simulink model "LKA"  (R2024a)
settings: Solver=ode1  StartTime=0.0  StopTime=70  FixedStep=1e-1  RelTol=1e-3
model workspace (MAT data in the model file):
  firstWarning = 1
  originalScenarioChecksum = '148AF3F4C6D12E297BC90CA3DB8BB877'
values from neighbouring files (symbols this model uses):
  dt = 0.1    [Parameters.m]
  Ki = 1    [Parameters.m]
  Kp = 1.1    [Parameters.m]
  L1 = 3.7    [Parameters.m]
  lane_width = 3.6    [Parameters.m]
  lr = 1.6    [Parameters.m]
  m = 1575    [Parameters.m]
  PredictionHorizon = 2    [Parameters.m]
  tau1 = 0.5    [Parameters.m]
  tau2 = 0.07    [Parameters.m]
undefined symbols (not defined in the file or in its folder): driving
libraries: drivingscenarioandsensors x2, simulink x2, simulink_extras x2, slpidlib x1, autolibshared x1
settings Model: Creator=apple  LastModifiedBy=apple
settings OptimizationCC: DefaultParameterBehavior=Inlined  UseDivisionForNetSlopeComputation=on  GainParamInheritBuiltInType=on  UseFloatMulNetSlope=on  InlineInvariantSignals=on  PassReuseOutputArgsAs=Individual arguments  ZeroExternalMemoryAtStartup=off  ZeroInternalMemoryAtStartup=off  NoFixptDivByZeroProtection=on  EfficientFloat2IntCast=on  LifeSpan=1  OptimizeBlockOrder=speed  DifferentSizesBufferReuse=on  EfficientTunableParamExpr=on
settings DebuggingCC: ParameterTunabilityLossMsg=error
settings HardwareCC: ProdBitPerLong=64  ProdLongLongMode=on  ProdHWDeviceType=Apple->ARM64
settings SFSimCC: MATLABDynamicMemAlloc=off
settings RTWCC: Description=Embedded Coder  SystemTargetFile=ert.tlc  TemplateMakefile=ert_default_tmf
settings CodeAppCC: ForceParamTrailComments=on  IgnoreCustomStorageClasses=off  OperatorAnnotations=on  SimulinkDataObjDesc=on  SFDataObjDesc=on  CustomSymbolStrGlobalVar=rt$N$M  CustomSymbolStrType=$N$M  CustomSymbolStrFcn=$N$M$F  CustomSymbolStrMacro=$N$M  InsertBlockDesc=on
settings ERTTargetCC: TargetLangStandard=C99 (ISO)  GenerateSampleERTMain=on  IncludeMdlTerminateFcn=off  CombineSignalStateStructs=on  SupportAbsoluteTime=off  SupportComplex=off  SupportContinuousTime=on  SupportNonInlinedSFcns=on  InlinedParameterPlacement=NonHierarchical  ERTCustomFileTemplate=example_file_process.tlc  ERTFilePackagingFormat=CompactWithDataFile
settings ConfigComp: DVTestSuiteOptimization=Auto  DVDetectOutOfBounds=on  DVModelReferenceHarness=on  DVHarnessSource=Signal Editor

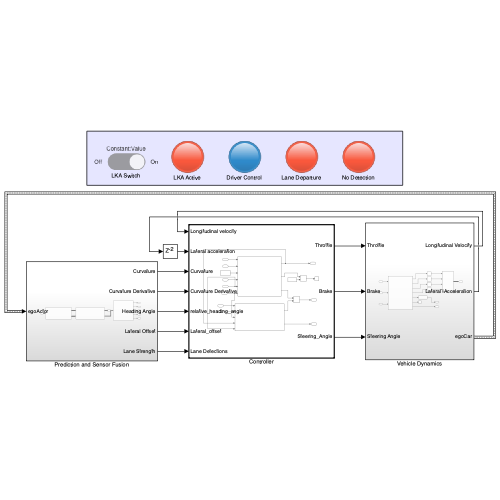
[thumbnail: Simulink's stored preview of the top-level diagram]
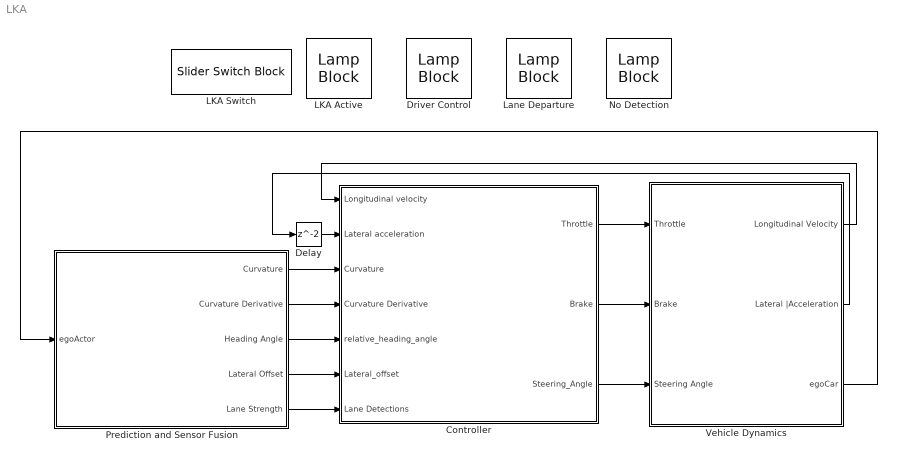
== system LKA ==
  Controller : Subsystem  TreatAsAtomicUnit=on
  Delay : Delay
  Driver Control : LampBlock  LabelPosition=Hide
  LKA Active : LampBlock  LabelPosition=Hide
  LKA Switch : SliderSwitchBlock
      settings: Values={{'Off', 'On'}, [0 1]}
  Lane Departure : LampBlock  LabelPosition=Hide
  No Detection : LampBlock  LabelPosition=Hide
  Prediction and Sensor Fusion : Subsystem
  Vehicle Dynamics : Subsystem
  wires:
  Vehicle Dynamics/3(egoCar) -> Prediction and Sensor Fusion/1(egoActor)
  Controller/1(Throttle) -> Vehicle Dynamics/1(Throttle)
  Controller/2(Brake) -> Vehicle Dynamics/2(Brake)
  Controller/3(Steering_Angle) -> Vehicle Dynamics/3(Steering Angle)
  Vehicle Dynamics/1(Longitudinal Velocity) -> Controller/1(Longitudinal velocity)
  Vehicle Dynamics/2(Lateral |Acceleration) -> Delay/1
  Prediction and Sensor Fusion/1(Curvature) -> Controller/3(Curvature)
  Prediction and Sensor Fusion/2(Curvature Derivative) -> Controller/4(Curvature Derivative)
  Prediction and Sensor Fusion/3(Heading Angle) -> Controller/5(relative_heading_angle)
  Prediction and Sensor Fusion/4(Lateral Offset) -> Controller/6(Lateral_offset)
  Prediction and Sensor Fusion/5(Lane Strength) -> Controller/7(Lane Detections)
  Delay/1 -> Controller/2(Lateral acceleration)

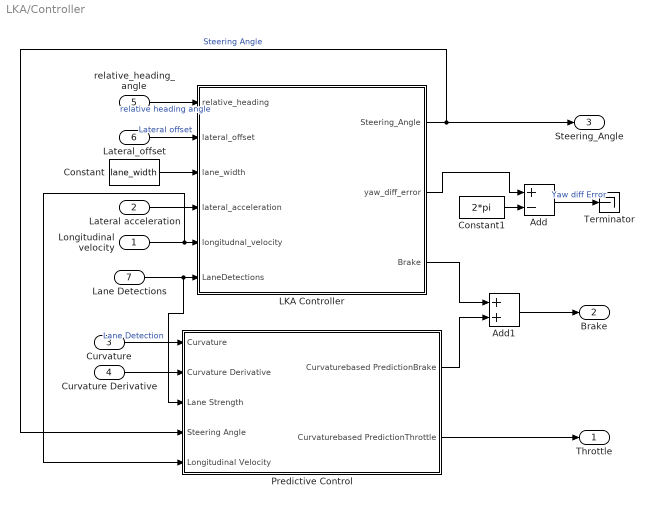
== system LKA/Controller ==
  Longitudinal velocity : Inport
  Lateral acceleration : Inport  Port=2
  Curvature : Inport  Port=3
  Curvature Derivative : Inport  Port=4
  relative_heading_angle : Inport  Port=5
  Lateral_offset : Inport  Port=6
  Lane Detections : Inport  Port=7
  Add : Sum  Inputs=+-
  Add1 : Sum
  Constant : Constant  Value=lane_width
  Constant1 : Constant  Value=2*pi
  LKA Controller : Subsystem
  Predictive Control : Subsystem
  Terminator : Terminator
  Throttle : Outport
  Brake : Outport  Port=2
  Steering_Angle : Outport  Port=3
  wires:
  Constant/1 -> LKA Controller/3(lane_width)
  Lane Detections/1 -> Predictive Control/3(Lane Strength), LKA Controller/6(LaneDetections)  "Lane Detection"
  Lateral acceleration/1 -> LKA Controller/4(lateral_acceleration)
  Lateral_offset/1 -> LKA Controller/2(lateral_offset)  "Lateral offset"
  relative_heading_angle/1 -> LKA Controller/1(relative_heading)  "relative heading angle"
  Longitudinal velocity/1 -> Predictive Control/5(Longitudinal Velocity), LKA Controller/5(longitudnal_velocity)
  LKA Controller/1(Steering_Angle) -> Steering_Angle/1, Predictive Control/4(Steering Angle)  "Steering Angle"
  LKA Controller/2(yaw_diff_error) -> Add/1
  Add/1 -> Terminator/1  "Yaw diff Error"
  Constant1/1 -> Add/2
  Curvature/1 -> Predictive Control/1(Curvature)
  Curvature Derivative/1 -> Predictive Control/2(Curvature Derivative)
  LKA Controller/3(Brake) -> Add1/1
  Predictive Control/1(Curvaturebased PredictionBrake) -> Add1/2
  Add1/1 -> Brake/1
  Predictive Control/2(Curvaturebased PredictionThrottle) -> Throttle/1

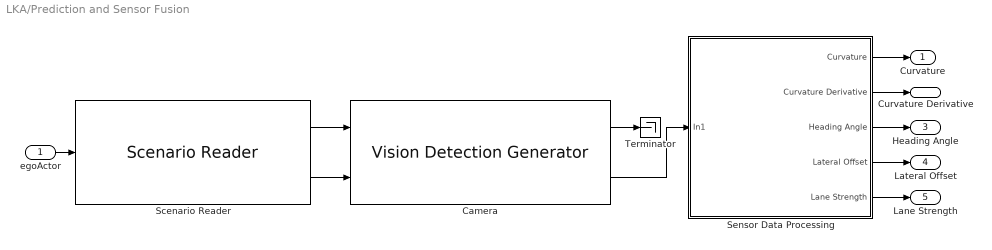
== system LKA/Prediction and Sensor Fusion ==
  egoActor : Inport
  Camera : drivingscenarioandsensors/Vision Detection Generator  SensorIndex=1  DetectorOutput=Lanes and objects  UpdateInterval=dt  LaneUpdateInterval=dt  SensorLocation=[1.9 0]  Height=1.1  Yaw=0  Pitch=10  Roll=0  BusNameSource=Auto  BusName=BusObjectDetections  BusName2Source=Property  BusName2=BusVision  MaxNumDetectionsSource=Property  MaxNumDetections=50  MaxNumLanesSource=Property  MaxNumLanes=2  DetectionCoordinates=Ego Cartesian  SimulateUsing=Interpreted execution  MaxRange=60  BoundingBoxAccuracy=5  ProcessNoiseIntensity=5  MaxSpeed=100  MaxAllowedOcclusion=0.5  MinObjectImageSize=[15 15]  DetectionProbability=0.9  FalsePositivesPerImage=0.1  MinLaneImageSize=[20 3]  LaneBoundaryAccuracy=3  HasNoise=on  InitialSeedSource=Repeatable  InitialSeed=0  UsedSeed=0  ActorProfilesSource=From Scenario Reader block  ActorProfilesParameters=driving.internal.ActorProfilesParameters  ActorProfilesExpression=[struct('ActorID',1,'ClassID',1,'Length',4.7,'Width',1.8,'Height',1.4,'OriginOffset',[-1.35 0 0],'MeshVertices',[3.7 0.9 0.857439446366782;3.7 -0.9 0.857439446366782;3.7 -0.9 0.314878892733564;3.7 0.9 0.314878892733564;3.7 0.9 0.857439446366782;2.525 0.9 0.993079584775086;2.525 -0.9 0.993079584775086;3.7 -0.9 0.857439446366782;1.82 0.72 1.4;0.41 0.72 1.4;0.41 -0.72 1.4;1.82 -0.72 1.4;-0.295 0.9 0.993079584775086;-1 0.9 0.857439446366782;-1 -0.9 0.857439446366782;-0.295 -0.9 0.993079584775086;3.7 0.9 0.857439446366782;3.7 0.9 0.314878892733564;2.525 0.9 0.314878892733564;2.525 0.9 0.993079584775086;2.525 0.9 0.993079584775086;2.525 0.9 0.314878892733564;-0.295 0.9 0.314878892733564;-0.295 0.9 0.993079584775086;-0.295 0.9 0.993079584775086;-0.295 0.9 0.314878892733564;-1 0.9 0.355570934256055;-1 0.9 0.857439446366782;2.525 0.9 0.993079584775086;-0.295 0.9 0.993079584775086;0.41 0.72 1.4;1.82 0.72 1.4;3.7 -0.9 0.857439446366782;3.7 -0.9 0.314878892733564;2.525 -0.9 0.314878892733564;2.525 -0.9 0.993079584775086;2.525 -0.9 0.993079584775086;2.525 -0.9 0.314878892733564;-0.295 -0.9 0.314878892733564;-0.295 -0.9 0.993079584775086;-0.295 -0.9 0.993079584775086;-0.295 -0.9 0.314878892733564;-1 -0.9 0.355570934256055;-1 -0.9 0.857439446366782;2.525 -0.9 0.993079584775086;-0.295 -0.9 0.993079584775086;0.41 -0.72 1.4;1.82 -0.72 1.4;-0.295 0.9 0.993079584775086;-0.295 -0.9 0.993079584775086;0.41 -0.72 1.4;0.41 0.72 1.4;2.525 -0.9 0.993079584775086;1.82 -0.72 1.4;1.82 0.72 1.4;2.525 0.9 0.993079584775086;-1 0.9 0.857439446366782;-1 0.9 0.355570934256055;-1 -0.9 0.355570934256055;-1 -0.9 0.857439446366782;3.7 0.9 0.314878892733564;3.7 -0.9 0.314878892733564;-0.295 -0.9 0.314878892733564;-0.295 0.9 0.314878892733564;-0.295 0.9 0.314878892733564;-1 0.9 0.355570934256055;-1 -0.9 0.355570934256055;-0.295 -0.9 0.314878892733564;0 -0.63 0;0 -0.87 0;0.191030206995054 -0.63 0.0601365173421445;0.191030206995054 -0.87 0.0601365173421445;0.309093367795925 -0.63 0.217575963708927;0.309093367795925 -0.87 0.217575963708927;0.309093367795925 -0.63 0.412181821758201;0.309093367795925 -0.87 0.412181821758201;0.191030206995054 -0.63 0.569621268124983;0.191030206995054 -0.87 0.569621268124983;0 -0.63 0.629757785467128;0 -0.87 0.629757785467128;-0.191030206995054 -0.63 0.569621268124983;-0.191030206995054 -0.87 0.569621268124983;-0.309093367795925 -0.63 0.412181821758201;-0.309093367795925 -0.87 0.412181821758201;-0.309093367795925 -0.63 0.217575963708927;-0.309093367795925 -0.87 0.217575963708927;-0.191030206995054 -0.63 0.0601365173421445;-0.191030206995054 -0.87 0.0601365173421445;0 -0.63 0;0 -0.87 0;0 -0.63 0;0.191030206995054 -0.63 0.0601365173421445;0.309093367795925 -0.63 0.217575963708927;0.309093367795925 -0.63 0.412181821758201;0.191030206995054 -0.63 0.569621268124983;0 -0.63 0.629757785467128;-0.191030206995054 -0.63 0.569621268124983;-0.309093367795925 -0.63 0.412181821758201;-0.309093367795925 -0.63 0.217575963708927;-0.191030206995054 -0.63 0.0601365173421445;0 -0.87 0;0.191030206995054 -0.87 0.0601365173421445;0.309093367795925 -0.87 0.217575963708927;0.309093367795925 -0.87 0.412181821758201;0.191030206995054 -0.87 0.569621268124983;0 -0.87 0.629757785467128;-0.191030206995054 -0.87 0.569621268124983;-0.309093367795925 -0.87 0.412181821758201;-0.309093367795925 -0.87 0.217575963708927;-0.191030206995054 -0.87 0.0601365173421445;0 0.87 0;0 0.63 0;0.191030206995054 0.87 0.0601365173421445;0.191030206995054 0.63 0.0601365173421445;0.309093367795925 0.87 0.217575963708927;0.309093367795925 0.63 0.217575963708927;0.309093367795925 0.87 0.412181821758201;0.309093367795925 0.63 0.412181821758201;0.191030206995054 0.87 0.569621268124983;0.191030206995054 0.63 0.569621268124983;0 0.87 0.629757785467128;0 0.63 0.629757785467128;-0.191030206995054 0.87 0.569621268124983;-0.191030206995054 0.63 0.569621268124983;-0.309093367795925 0.87 0.412181821758201;-0.309093367795925 0.63 0.412181821758201;-0.309093367795925 0.87 0.217575963708927;-0.309093367795925 0.63 0.217575963708927;-0.191030206995054 0.87 0.0601365173421445;-0.191030206995054 0.63 0.0601365173421445;0 ...(+3718 chars)],'MeshFaces',[1 2 3;3 4 1;5 6 7;7 8 5;9 10 11;11 12 9;13 14 15;15 16 13;17 18 19;19 20 17;21 22 23;23 24 21;25 26 27;27 28 25;29 30 31;31 32 29;33 34 35;35 36 33;37 38 39;39 40 37;41 42 43;43 44 41;45 46 47;47 48 45;49 50 51;51 52 49;53 54 55;55 56 53;57 58 59;59 60 57;61 62 63;63 64 61;65 66 67;67 68 65;69 71 72;72 70 69;71 73 74;74 72 71;73 75 76;76 74 73;75 77 78;78 76 75;77 79 80;80 78 77;79 81 82;82 80 79;81 83 84;84 82 81;83 85 86;86 84 83;85 87 88;88 86 85;87 89 90;90 88 87;91 92 93;91 93 94;91 94 95;91 95 96;91 96 97;91 97 98;91 98 99;91 99 100;101 102 103;101 103 104;101 104 105;101 105 106;101 106 107;101 107 108;101 108 109;101 109 110;111 113 114;114 112 111;113 115 116;116 114 113;115 117 118;118 116 115;117 119 120;120 118 117;119 121 122;122 120 119;121 123 124;124 122 121;123 125 126;126 124 123;125 127 128;128 126 125;127 129 130;130 128 127;129 131 132;132 130 129;133 134 135;133 135 136;133 136 137;133 137 138;133 138 139;133 139 140;133 140 141;133 141 142;143 144 145;143 145 146;143 146 147;143 147 148;143 148 149;143 149 150;143 150 151;143 151 152;153 155 156;156 154 153;155 157 158;158 156 155;157 159 160;160 158 157;159 161 162;162 160 159;161 163 164;164 162 161;163 165 166;166 164 163;165 167 168;168 166 165;167 169 170;170 168 167;169 171 172;172 170 169;171 173 174;174 172 171;175 176 177;175 177 178;175 178 179;175 179 180;175 180 181;175 181 182;175 182 183;175 183 184;185 186 187;185 187 188;185 188 189;185 189 190;185 190 191;185 191 192;185 192 193;185 193 194;195 197 198;198 196 195;197 199 200;200 198 197;199 201 202;202 200 199;201 203 204;204 202 201;203 205 206;206 204 203;205 207 208;208 206 205;207 209 210;210 208 207;209 211 212;212 210 209;211 213 214;214 212 211;213 215 216;216 214 213;217 218 219;217 219 220;217 220 221;217 221 222;217 222 223;217 223 224;217 224 225;217 225 226;227 228 229;227 229 230;227 230 231;227 231 232;227 232 233;227 233 234;227 234 235;227 235 236],'RCSPattern',[10 10;10 10],'RCSAzimuthAngles',[-180 180],'RCSElevationAngles',[-90 90])]  Intrinsics=driving.internal.cameraIntrinsics('FocalLength',[340 720],'PrincipalPoint',[640 480],'ImageSize',[960 1280],'RadialDistortion',[0 0],'TangentialDistortion',[0 0],'Skew',0)
  Scenario Reader : drivingscenarioandsensors/Scenario Reader  ScenarioSource=From file  ScenarioFileName=/Users/apple/Documents/VCSE/Practice/test_scenario_1.mat  ScenarioVariableName=scenario  OutputCoordinateSystem=Vehicle coordinates  EgoVehicleSource=Input port  EgoVehicleActorID=1  OrientVehiclesOnRoad=off  OutputEgoVehiclePose=off  OutputEgoVehicleState=off  SampleTime=dt  LaneBoundaryOutput=Ego vehicle lane boundaries  LaneBoundaryDistance=0:0.5:60  LaneBoundaryLocation=Inner edge of lane markings  BusNameSource=Auto  BusName=BusActors  BusNumActorsSource=Scenario  BusNumActors=100  BusName2Source=Auto  BusName2=BusLaneBoundaries  BusNumLaneBoundariesSource=Scenario  BusNumLaneBoundaries=10  BusName3Source=Auto  BusName3=BusEgoActor  BusName4Source=Auto  BusName4=BusEgoState  ShowCoordinateLabels=on  SimulateUsing=Interpreted execution
  Sensor Data Processing : Subsystem
  Terminator : Terminator
  Curvature : Outport
  Curvature Derivative : Outport  Port=2
  Heading Angle : Outport  Port=3
  Lateral Offset : Outport  Port=4
  Lane Strength : Outport  Port=5
  wires:
  Camera/1 -> Terminator/1
  Scenario Reader/2 -> Camera/2
  Camera/2 -> Sensor Data Processing/1(In1)
  egoActor/1 -> Scenario Reader/1
  Scenario Reader/1 -> Camera/1
  Sensor Data Processing/2(Curvature Derivative) -> Curvature Derivative/1
  Sensor Data Processing/1(Curvature) -> Curvature/1
  Sensor Data Processing/3(Heading Angle) -> Heading Angle/1
  Sensor Data Processing/4(Lateral Offset) -> Lateral Offset/1
  Sensor Data Processing/5(Lane Strength) -> Lane Strength/1

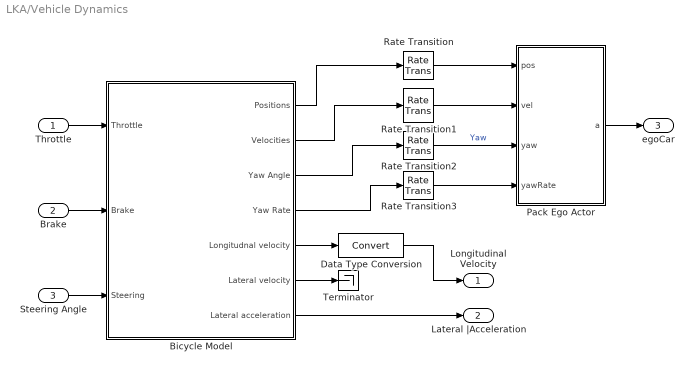
== system LKA/Vehicle Dynamics ==
  Throttle : Inport
  Brake : Inport  Port=2
  Steering Angle : Inport  Port=3
  Bicycle Model : Subsystem
  Data Type Conversion : DataTypeConversion  SaturateOnIntegerOverflow=off  RndMeth=Floor
  Pack Ego Actor : MATLAB Function  TreatAsAtomicUnit=on
  Rate Transition{,1..3} (4 alike) : RateTransition  OutPortSampleTime=Ts
  Terminator : Terminator
  Longitudinal Velocity : Outport
  Lateral |Acceleration : Outport  Port=2
  egoCar : Outport  Port=3
  wires:
  Bicycle Model/1(Positions) -> Rate Transition/1
  Bicycle Model/2(Velocities) -> Rate Transition1/1
  Bicycle Model/3(Yaw Angle) -> Rate Transition2/1
  Bicycle Model/4(Yaw Rate) -> Rate Transition3/1
  Bicycle Model/5(Longitudnal velocity) -> Data Type Conversion/1
  Data Type Conversion/1 -> Longitudinal Velocity/1
  Bicycle Model/6(Lateral velocity) -> Terminator/1
  Bicycle Model/7(Lateral acceleration) -> Lateral |Acceleration/1
  Steering Angle/1 -> Bicycle Model/3(Steering)
  Brake/1 -> Bicycle Model/2(Brake)
  Throttle/1 -> Bicycle Model/1(Throttle)
  Pack Ego Actor/1(a) -> egoCar/1
  Rate Transition/1 -> Pack Ego Actor/1(pos)
  Rate Transition1/1 -> Pack Ego Actor/2(vel)
  Rate Transition2/1 -> Pack Ego Actor/3(yaw)  "Yaw"
  Rate Transition3/1 -> Pack Ego Actor/4(yawRate)

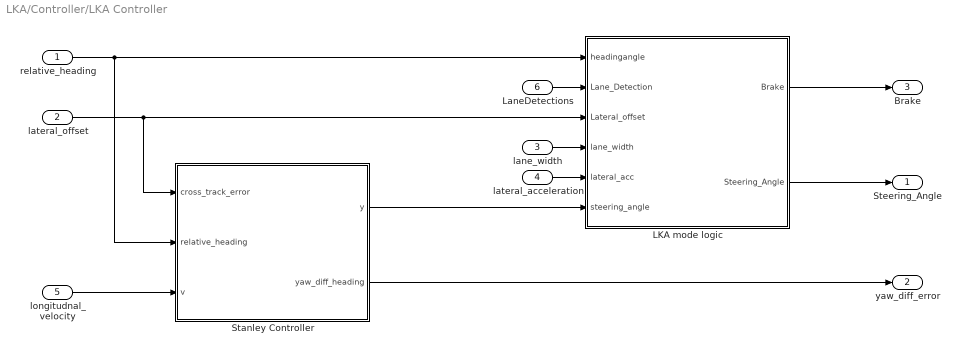
== system LKA/Controller/LKA Controller ==
  relative_heading : Inport
  lateral_offset : Inport  Port=2
  lane_width : Inport  Port=3
  lateral_acceleration : Inport  Port=4
  longitudnal_velocity : Inport  Port=5
  LaneDetections : Inport  Port=6
  LKA mode logic : Subsystem
  Stanley Controller : MATLAB Function  TreatAsAtomicUnit=on
  Steering_Angle : Outport
  yaw_diff_error : Outport  Port=2
  Brake : Outport  Port=3
  wires:
  LKA mode logic/2(Steering_Angle) -> Steering_Angle/1
  LKA mode logic/1(Brake) -> Brake/1
  lateral_acceleration/1 -> LKA mode logic/5(lateral_acc)
  longitudnal_velocity/1 -> Stanley Controller/3(v)
  lateral_offset/1 -> LKA mode logic/3(Lateral_offset), Stanley Controller/1(cross_track_error)
  lane_width/1 -> LKA mode logic/4(lane_width)
  Stanley Controller/1(y) -> LKA mode logic/6(steering_angle)
  LaneDetections/1 -> LKA mode logic/2(Lane_Detection)
  Stanley Controller/2(yaw_diff_heading) -> yaw_diff_error/1
  relative_heading/1 -> LKA mode logic/1(headingangle), Stanley Controller/2(relative_heading)

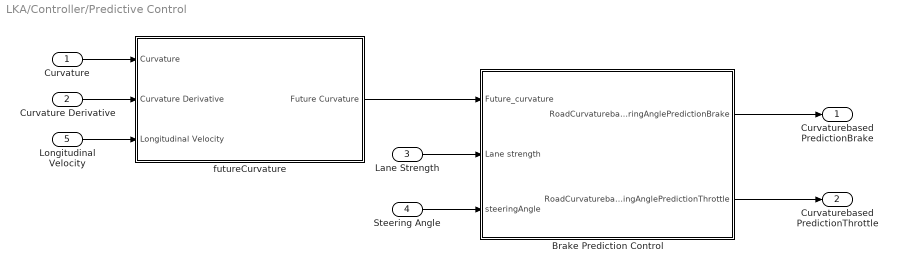
== system LKA/Controller/Predictive Control ==
  Curvature : Inport
  Curvature Derivative : Inport  Port=2
  Lane Strength : Inport  Port=3
  Steering Angle : Inport  Port=4
  Longitudinal Velocity : Inport  Port=5
  Brake Prediction Control : Subsystem
  futureCurvature : Subsystem
  Curvaturebased PredictionBrake : Outport
  Curvaturebased PredictionThrottle : Outport  Port=2
  wires:
  Curvature/1 -> futureCurvature/1(Curvature)
  Curvature Derivative/1 -> futureCurvature/2(Curvature Derivative)
  Longitudinal Velocity/1 -> futureCurvature/3(Longitudinal Velocity)
  futureCurvature/1(Future Curvature) -> Brake Prediction Control/1(Future_curvature)
  Lane Strength/1 -> Brake Prediction Control/2(Lane strength)
  Steering Angle/1 -> Brake Prediction Control/3(steeringAngle)
  Brake Prediction Control/2(RoadCurvaturebased SteeringAnglePredictionThrottle) -> Curvaturebased PredictionThrottle/1
  Brake Prediction Control/1(RoadCurvaturebased SteeringAnglePredictionBrake) -> Curvaturebased PredictionBrake/1

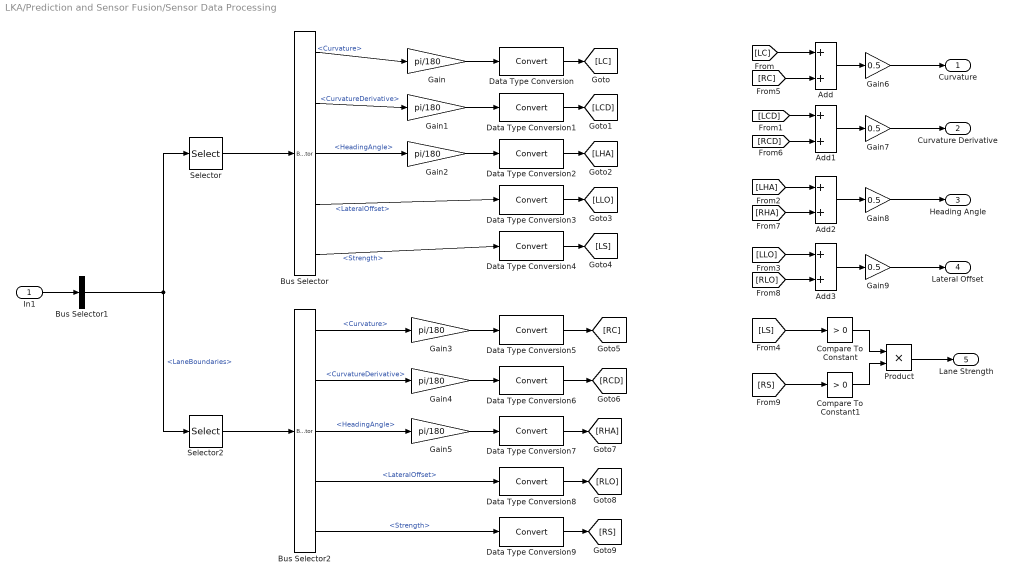
== system LKA/Prediction and Sensor Fusion/Sensor Data Processing ==
  In1 : Inport
  Add{,1..3} (4 alike) : Sum
  Bus Selector : BusSelector  OutputSignals=Curvature,CurvatureDerivative,HeadingAngle,LateralOffset,Strength
  Bus Selector1 : BusSelector  OutputSignals=LaneBoundaries
  Bus Selector2 : BusSelector  OutputSignals=Curvature,CurvatureDerivative,HeadingAngle,LateralOffset,Strength
  Compare To Constant : simulink/Logic and Bit Operations/Compare To Constant  relop=>  const=0  OutDataTypeStr=boolean
  Compare To Constant1 : simulink/Logic and Bit Operations/Compare To Constant  relop=>  const=0  OutDataTypeStr=boolean
  Data Type Conversion{,1..9} (10 alike) : DataTypeConversion  SaturateOnIntegerOverflow=off  RndMeth=Floor
  Gain{,1..5} (6 alike) : Gain  Gain=pi/180
  Gain{6..9} (4 alike) : Gain  Gain=0.5
  Product : Product
  Selector : Selector  InputPortWidth=2  IndexOptions=Index vector (dialog)  Indices=1  OutputSizes=1
  Selector2 : Selector  InputPortWidth=2  IndexOptions=Index vector (dialog)  Indices=2  OutputSizes=1
  Curvature : Outport
  Curvature Derivative : Outport  Port=2
  Heading Angle : Outport  Port=3
  Lateral Offset : Outport  Port=4
  Lane Strength : Outport  Port=5
  wires:
  In1/1 -> Bus Selector1/1
  Bus Selector1/1 -> Selector2/1, Selector/1  "<LaneBoundaries>"
  Selector2/1 -> Bus Selector2/1
  Selector/1 -> Bus Selector/1
  Bus Selector/1 -> Gain/1  "<Curvature>"
  Bus Selector/2 -> Gain1/1  "<CurvatureDerivative>"
  Bus Selector/3 -> Gain2/1  "<HeadingAngle>"
  Bus Selector/4 -> Data Type Conversion3/1  "<LateralOffset>"
  Bus Selector/5 -> Data Type Conversion4/1  "<Strength>"
  Bus Selector2/1 -> Gain3/1  "<Curvature>"
  Gain/1 -> Data Type Conversion/1
  Gain1/1 -> Data Type Conversion1/1
  Gain2/1 -> Data Type Conversion2/1
  Gain4/1 -> Data Type Conversion6/1
  Gain5/1 -> Data Type Conversion7/1
  Bus Selector2/5 -> Data Type Conversion9/1  "<Strength>"
  Gain3/1 -> Data Type Conversion5/1
  Bus Selector2/4 -> Data Type Conversion8/1  "<LateralOffset>"
  Bus Selector2/2 -> Gain4/1  "<CurvatureDerivative>"
  Bus Selector2/3 -> Gain5/1  "<HeadingAngle>"
  Data Type Conversion/1 -> [LC]
  Data Type Conversion2/1 -> [LHA]
  Data Type Conversion1/1 -> [LCD]
  Data Type Conversion3/1 -> [LLO]
  Data Type Conversion4/1 -> [LS]
  Data Type Conversion5/1 -> [RC]
  Data Type Conversion6/1 -> [RCD]
  Data Type Conversion7/1 -> [RHA]
  Data Type Conversion8/1 -> [RLO]
  Data Type Conversion9/1 -> [RS]
  [LC] -> Add/1
  [RC] -> Add/2
  Add/1 -> Gain6/1
  Gain6/1 -> Curvature/1
  Gain7/1 -> Curvature Derivative/1
  Add1/1 -> Gain7/1
  [LCD] -> Add1/1
  [RCD] -> Add1/2
  Gain8/1 -> Heading Angle/1
  Add2/1 -> Gain8/1
  [LHA] -> Add2/1
  [RHA] -> Add2/2
  Gain9/1 -> Lateral Offset/1
  Add3/1 -> Gain9/1
  [LLO] -> Add3/1
  [RLO] -> Add3/2
  [LS] -> Compare To Constant/1
  [RS] -> Compare To Constant1/1
  Compare To Constant1/1 -> Product/2
  Compare To Constant/1 -> Product/1
  Product/1 -> Lane Strength/1

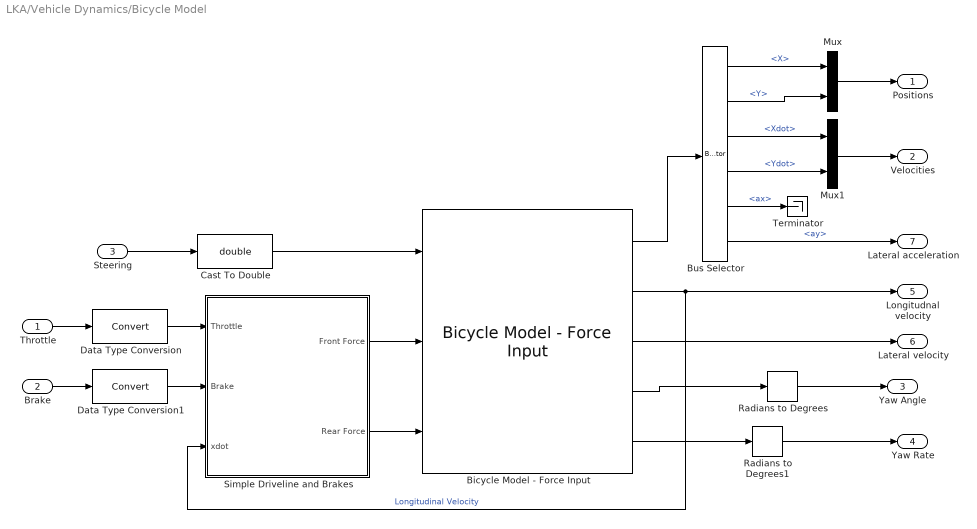
== system LKA/Vehicle Dynamics/Bicycle Model ==
  Throttle : Inport
  Brake : Inport  Port=2
  Steering : Inport  Port=3
  Bicycle Model - Force Input : autolibshared/Bicycle Model - Force Input  trackMode=Single (bicycle)  inputMode=External longitudinal forces  frontSteerMode=on  rearSteerMode=off  windMode=off  muMode=off  extFMode=off  extMMode=off  aMode=3  NF=2  NR=2  m=m  a=lf  b=lr  h=0.35  X_o=x0_ego  xdot_o=v0_ego  CalphaMode=off  sigmaMode=on  w=[1.4,1.4]  Cy_f=Cf  Cy_r=Cr  sigma_f=.1  sigma_r=.1  alpha_f_brk=[-.1 .1]  Cy_f_data=[-9e3 9e3]  alpha_r_brk=[-.1 .1]  Cy_r_data=[-9e3 9e3]  Y_o=y0_ego  ydot_o=0  Izz=Iz  psi_o=0  r_o=yaw0_ego  Af=0  Cd=.3  Cl=.1  Cpm=.1  beta_w=[0:0.01:0.3]  Cs=[0:0.03:0.9]  Cym=[0:0.01:0.3]  Pabs=101325  Tair=273  g=9.81  mu=1  xdot_tol=.01  Fznom=5000  Fxtire_sat=1e6  Fytire_sat=1e6  longOff=0  latOff=0  vertOff=0
      settings: LibrarySourceBlock=drivingscenarioandsensors/Bicycle Model - Force Input
  Bus Selector : BusSelector  OutputSignals=InertFrm.FrntAxl.Disp.X,InertFrm.FrntAxl.Disp.Y,InertFrm.FrntAxl.Vel.Xdot,InertFrm.FrntAxl.Vel.Ydot,BdyFrm.Cg.Acc.ax,BdyFrm.Cg.Acc.ay
  Cast To Double : DataTypeConversion  OutDataTypeStr=double  SaturateOnIntegerOverflow=off  RndMeth=Floor
  Data Type Conversion : DataTypeConversion  SaturateOnIntegerOverflow=off  RndMeth=Floor
  Data Type Conversion1 : DataTypeConversion  SaturateOnIntegerOverflow=off  RndMeth=Floor
  Mux : Mux  Inputs=2
  Mux1 : Mux  Inputs=2
  Radians to Degrees : simulink_extras/Transformations/Radians to Degrees
  Radians to Degrees1 : simulink_extras/Transformations/Radians to Degrees
  Simple Driveline and Brakes : Subsystem
  Terminator : Terminator
  Positions : Outport
  Velocities : Outport  Port=2
  Yaw Angle : Outport  Port=3
  Yaw Rate : Outport  Port=4
  Longitudnal velocity : Outport  Port=5
  Lateral velocity : Outport  Port=6
  Lateral acceleration : Outport  Port=7
  wires:
  Steering/1 -> Cast To Double/1
  Cast To Double/1 -> Bicycle Model - Force Input/1
  Simple Driveline and Brakes/1(Front Force) -> Bicycle Model - Force Input/2
  Simple Driveline and Brakes/2(Rear Force) -> Bicycle Model - Force Input/3
  Throttle/1 -> Data Type Conversion/1
  Brake/1 -> Data Type Conversion1/1
  Data Type Conversion1/1 -> Simple Driveline and Brakes/2(Brake)
  Data Type Conversion/1 -> Simple Driveline and Brakes/1(Throttle)
  Bicycle Model - Force Input/1 -> Bus Selector/1
  Bus Selector/4 -> Mux1/2  "<Ydot>"
  Bus Selector/6 -> Lateral acceleration/1  "<ay>"
  Bus Selector/5 -> Terminator/1  "<ax>"
  Bus Selector/3 -> Mux1/1  "<Xdot>"
  Bus Selector/2 -> Mux/2  "<Y>"
  Bus Selector/1 -> Mux/1  "<X>"
  Mux/1 -> Positions/1
  Mux1/1 -> Velocities/1
  Bicycle Model - Force Input/2 -> Simple Driveline and Brakes/3(xdot), Longitudnal velocity/1  "Longitudinal Velocity"
  Bicycle Model - Force Input/3 -> Lateral velocity/1
  Bicycle Model - Force Input/5 -> Radians to Degrees1/1
  Radians to Degrees1/1 -> Yaw Rate/1
  Bicycle Model - Force Input/4 -> Radians to Degrees/1
  Radians to Degrees/1 -> Yaw Angle/1

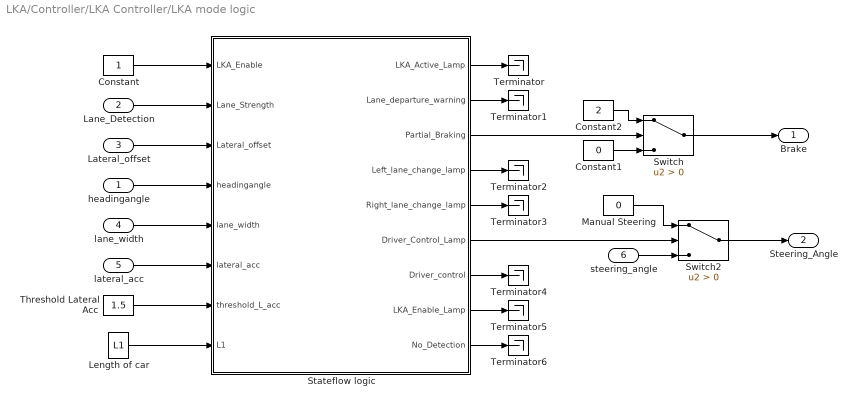
== system LKA/Controller/LKA Controller/LKA mode logic ==
  headingangle : Inport
  Lane_Detection : Inport  Port=2
  Lateral_offset : Inport  Port=3
  lane_width : Inport  Port=4
  lateral_acc : Inport  Port=5
  steering_angle : Inport  Port=6
  Constant : Constant
  Constant1 : Constant  Value=0
  Constant2 : Constant  Value=2
  Length of car : Constant  Value=L1
  Manual Steering : Constant  Value=0
  Stateflow logic : Stateflow chart  TreatAsAtomicUnit=on
  Switch : Switch  Criteria=u2 > Threshold  SaturateOnIntegerOverflow=off  InputSameDT=off
  Switch2 : Switch  Criteria=u2 > Threshold  SaturateOnIntegerOverflow=off  InputSameDT=off
  Terminator{,1..6} (7 alike) : Terminator
  Threshold Lateral Acc : Constant  Value=1.5
  Brake : Outport
  Steering_Angle : Outport  Port=2
  wires:
  Constant/1 -> Stateflow logic/1(LKA_Enable)
  Lateral_offset/1 -> Stateflow logic/3(Lateral_offset)
  Lane_Detection/1 -> Stateflow logic/2(Lane_Strength)
  lane_width/1 -> Stateflow logic/5(lane_width)
  lateral_acc/1 -> Stateflow logic/6(lateral_acc)
  Threshold Lateral Acc/1 -> Stateflow logic/7(threshold_L_acc)
  Length of car/1 -> Stateflow logic/8(L1)
  headingangle/1 -> Stateflow logic/4(headingangle)
  Stateflow logic/3(Partial_Braking) -> Switch/2
  Constant1/1 -> Switch/3
  Switch/1 -> Brake/1
  Constant2/1 -> Switch/1
  Stateflow logic/6(Driver_Control_Lamp) -> Switch2/2
  Manual Steering/1 -> Switch2/1
  steering_angle/1 -> Switch2/3
  Switch2/1 -> Steering_Angle/1
  Stateflow logic/9(No_Detection) -> Terminator6/1
  Stateflow logic/8(LKA_Enable_Lamp) -> Terminator5/1
  Stateflow logic/4(Left_lane_change_lamp) -> Terminator2/1
  Stateflow logic/1(LKA_Active_Lamp) -> Terminator/1
  Stateflow logic/2(Lane_departure_warning) -> Terminator1/1
  Stateflow logic/5(Right_lane_change_lamp) -> Terminator3/1
  Stateflow logic/7(Driver_control) -> Terminator4/1

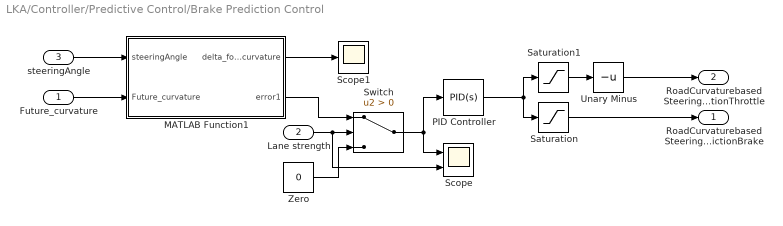
== system LKA/Controller/Predictive Control/Brake Prediction Control ==
  Future_curvature : Inport
  Lane strength : Inport  Port=2
  steeringAngle : Inport  Port=3
  MATLAB Function1 : MATLAB Function  TreatAsAtomicUnit=on
  PID Controller : slpidlib/PID Controller  Controller=PID  Form=Parallel  TimeDomain=Continuous-time  UseExternalTs=off  SampleTime=-1  IntegratorMethod=Forward Euler  FilterMethod=Forward Euler  ControllerParametersSource=internal  P=Kp  I=Ki  UseKiTs=off  D=0  UseExternalDerivativeSource=off  N=100  UseFilter=on  TunerSelectOption=Transfer Function Based (PID Tuner App)  InitialConditionSource=internal  InitialConditionForIntegrator=0  InitialConditionForFilter=0  DifferentiatorICPrevScaledInput=0  ExternalReset=none  TrackingMode=off  Kt=1  LimitOutput=on  SatLimitsSource=internal  UpperSaturationLimit=inf  LowerSaturationLimit=-inf  LinearizeAsGain=on  AntiWindupMode=none  Kb=1  LimitIntegrator=off  UpperIntegratorSaturationLimit=inf  LowerIntegratorSaturationLimit=-inf  POutMin=[]  POutMax=[]  IOutMin=[]  IOutMax=[]  DOutMin=[]  DOutMax=[]  NOutMin=[]  NOutMax=[]  SumOutMin=[]  SumOutMax=[]  SaturationOutMin=[]  SaturationOutMax=[]  PParamMin=[]  PParamMax=[]  IParamMin=[]  IParamMax=[]  DParamMin=[]  DParamMax=[]  NParamMin=[]  NParamMax=[]  KbParamMin=[]  KbParamMax=[]  KtParamMin=[]  KtParamMax=[]  KbOutMin=[]  KbOutMax=[]  KtOutMin=[]  KtOutMax=[]  IntegratorOutMin=[]  IntegratorOutMax=[]  FilterOutMin=[]  FilterOutMax=[]  SumI1OutMin=[]  SumI1OutMax=[]  SumI2OutMin=[]  SumI2OutMax=[]  SumI3OutMin=[]  SumI3OutMax=[]  SumI4OutMin=[]  SumI4OutMax=[]  SumDOutMin=[]  SumDOutMax=[]  DifferentiatorOutMin=[]  DifferentiatorOutMax=[]  FilterDiffOutCoefMin=[]  FilterDiffOutCoefMax=[]  ReciprocalOutMin=[]  ReciprocalOutMax=[]  SumDenOutMin=[]  SumDenOutMax=[]  SumNumOutMin=[]  SumNumOutMax=[]  DivideOutMin=[]  DivideOutMax=[]  UdiffTsProdOutMin=[]  UdiffTsProdOutMax=[]  NTsProdOutMin=[]  NTsProdOutMax=[]  UintegralTsProdOutMin=[]  UintegralTsProdOutMax=[]  UngainTsProdOutMin=[]  UngainTsProdOutMax=[]  ClampingZeroOutDataTypeStr=Inherit: Inherit via back propagation  ClampingZeroOutMin=[]  ClampingZeroOutMax=[]  FilterDenConstantOutDataTypeStr=Inherit: Inherit via back propagation  FilterDenConstantOutMin=[]  FilterDenConstantOutMax=[]  PCopyOutDataTypeStr=Inherit: Inherit via back propagation  PCopyOutMin=[]  PCopyOutMax=[]  NCopyOutDataTypeStr=Inherit: Inherit via back propagation  NCopyOutMin=[]  NCopyOutMax=[]  IntegratorContinuousStateAttributes=''  IntegratorStateMustResolveToSignalObject=off  IntegratorRTWStateStorageClass=Auto  FilterContinuousStateAttributes=''  FilterStateMustResolveToSignalObject=off  FilterRTWStateStorageClass=Auto  ParallelPVariant=InternalParameters  IdealPVariant=Disabled  IVariant=InternalParameters  DVariant=InternalParameters  IntegratorVariant=Continuous  SatVariant=Enabled  AWVariant=Passthrough  PCopyVariant=Disabled  TRVariant=Disabled  FdbkBlocksVariant=Forward  IdealPFdbkVariant=Disabled  SatFdbkVariant=Disabled  DerivativeFilterVariant=ContFilter  NVariant=InternalParameters  NCopyVariant=Disabled  FilterICVariant=InternalICsFilter  IntegratorICVariant=InternalICs  ExternalResetVariant=Disabled  TRSumVariant=Passthrough  SumFdbkVariant=Disabled  SumVariant=Sum_PID  TsampFilterVariant=InternalTs  TsampNgainVariant=Passthrough  TsampIntegralVariant=Disabled_SignalSpec  ExternalSaturationOutDataTypeStr=Inherit: Same as second input  DerivativeSourceVariant=ErrorSignal
  Saturation : Saturate  UpperLimit=inf  LowerLimit=0
  Saturation1 : Saturate  UpperLimit=0  LowerLimit=-inf
  Scope : Scope  NumInputPorts=2
  Scope1 : Scope
  Switch : Switch  Criteria=u2 > Threshold  SaturateOnIntegerOverflow=off  InputSameDT=off
  Unary Minus : UnaryMinus
  Zero : Constant  Value=0  OutDataTypeStr=Inherit: Inherit via back propagation
  RoadCurvaturebased SteeringAnglePredictionBrake : Outport
  RoadCurvaturebased SteeringAnglePredictionThrottle : Outport  Port=2
  wires:
  Future_curvature/1 -> MATLAB Function1/2(Future_curvature)
  Lane strength/1 -> Scope/2, Switch/2
  Saturation1/1 -> Unary Minus/1
  Saturation/1 -> RoadCurvaturebased SteeringAnglePredictionBrake/1
  PID Controller/1 -> Saturation1/1, Saturation/1
  Unary Minus/1 -> RoadCurvaturebased SteeringAnglePredictionThrottle/1
  steeringAngle/1 -> MATLAB Function1/1(steeringAngle)
  MATLAB Function1/1(delta_for_curvature) -> Scope1/1
  Zero/1 -> Switch/3
  Switch/1 -> Scope/1, PID Controller/1
  MATLAB Function1/2(error1) -> Switch/1

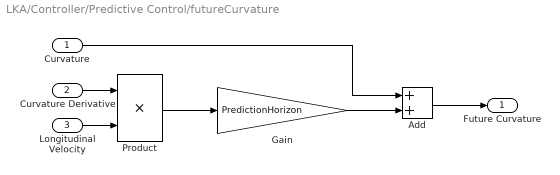
== system LKA/Controller/Predictive Control/futureCurvature ==
  Curvature : Inport
  Curvature Derivative : Inport  Port=2
  Longitudinal Velocity : Inport  Port=3
  Add : Sum
  Gain : Gain  Gain=PredictionHorizon
  Product : Product
  Future Curvature : Outport
  wires:
  Curvature/1 -> Add/1
  Curvature Derivative/1 -> Product/1
  Longitudinal Velocity/1 -> Product/2
  Product/1 -> Gain/1
  Gain/1 -> Add/2
  Add/1 -> Future Curvature/1

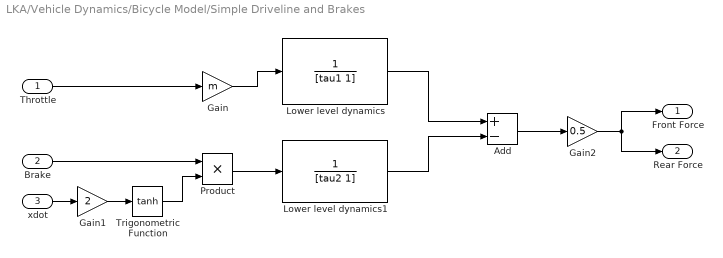
== system LKA/Vehicle Dynamics/Bicycle Model/Simple Driveline and Brakes ==
  Throttle : Inport
  Brake : Inport  Port=2
  xdot : Inport  Port=3
  Add : Sum  Inputs=+-
  Gain : Gain  Gain=m
  Gain1 : Gain  Gain=2
  Gain2 : Gain  Gain=0.5
  Lower level dynamics : TransferFcn  Denominator=[tau1 1]
  Lower level dynamics1 : TransferFcn  Denominator=[tau2 1]
  Product : Product
  Trigonometric Function : Trigonometry  Operator=tanh
  Front Force : Outport
  Rear Force : Outport  Port=2
  wires:
  Gain2/1 -> Front Force/1, Rear Force/1
  Add/1 -> Gain2/1
  Lower level dynamics/1 -> Add/1
  Lower level dynamics1/1 -> Add/2
  Gain/1 -> Lower level dynamics/1
  Trigonometric Function/1 -> Product/2
  Brake/1 -> Product/1
  xdot/1 -> Gain1/1
  Gain1/1 -> Trigonometric Function/1
  Product/1 -> Lower level dynamics1/1
  Throttle/1 -> Gain/1

== matlab function LKA/Controller/LKA Controller/Stanley Controller ==
  data: cross_track_error input; y output; relative_heading input; v input; yaw_diff_heading output
function [y,yaw_diff_heading] = fcn(cross_track_error, relative_heading,v)
   
% Use stanley controller for lateral control
    k_e = 3;
    k_s=0.01;
    steering_max_limit=1.22;
    steering_min_limit=-1.22;
   
    yaw_diff_heading=relative_heading;% - (yaw*pi/180); 
    if (yaw_diff_heading > pi)
        while(yaw_diff_heading>pi)
             yaw_diff_heading =yaw_diff_heading - 2 * pi;
        end
    else
         while(yaw_diff_heading<pi)
             yaw_diff_heading =yaw_diff_heading + 2 * pi;
         end
    end

   e=cross_track_error;

   yaw_diff_crosstrack = atan2(k_e .* e , (v+k_s));

   steer_expect = yaw_diff_crosstrack + yaw_diff_heading;
   if (steer_expect > pi)
        while(steer_expect>pi)
             steer_expect =steer_expect- 2 * pi;
        end
   else
       while(steer_expect<pi)
             steer_expect =steer_expect + 2 * pi;
       end
   end

  steer_expect1 = min(steering_max_limit, steer_expect);
  steer_expect2 = max(steering_min_limit, steer_expect1);

%update
 steer_output = steer_expect2;
 y=steer_output;
end

== matlab function LKA/Controller/Predictive Control/Brake Prediction Control/MATLAB Function1 ==
  data: steeringAngle input; Future_curvature input; delta_for_curvature output; error1 output
function [delta_for_curvature, error1] = fcn(steeringAngle, Future_curvature)
lf      = 1.2;      
lr      = 1.6;   

delta_for_curvature=atan((lf+lr)*Future_curvature);
error1=delta_for_curvature-steeringAngle;
%{
steering_limit=1.22;
error=delta_for_curvature-0.05*steering_limit;
if error>0
    error1=delta_for_curvature-steeringAngle;
else
    error1=0;
end
%}

== matlab function LKA/Vehicle Dynamics/Pack Ego Actor ==
  data: pos input; a output Bus: BusActors1Actors size=1; vel input; yaw input; yawRate input
function a = packEgo(pos,vel,yaw,yawRate)
% Pack ego information into a single ego actor bus
%
% Imoprtant note:
% Output is a bus of type BusActorsActors. This is the same bus used by the
% Scenario Reader to output an individual actor. If you change the
% output bus name of Scenario Reader change the output bus name here
% as well by clicking on 'Edit Data' in the menu above.

a = struct(...
    'ActorID',1,...
    'Position', [pos(1) pos(2) 0], ...
    'Velocity', [vel(1) vel(2) 0], ...
    'Roll', 0, ...
    'Pitch', 0, ...
    'Yaw', yaw, ...
    'AngularVelocity', [0 0 yawRate]);

== stateflow chart LKA/Controller/LKA Controller/LKA mode logic/Stateflow logic ==
  state LKA_Initating
    entry:
    Driver_Control_Lamp=1;
    LKA_Enable_Lamp=1;
    LKA_Active_Lamp=0;
    Partial_Braking=0;
    Left_lane_change_lamp=0;
    Right_lane_change_lamp=0;
    during:
    Driver_control=1;
  state Driver_control
    entry:
    Driver_Control_Lamp=1;
    LKA_Enable_Lamp=0;
    LKA_Active_Lamp=0;
    Partial_Braking=0;
    during:
    Driver_control=1;
  state LKA_active
    entry:
    Driver_Control_Lamp=0;
    LKA_Enable_Lamp=1;
    LKA_Active_Lamp=1;
    Partial_Braking=0;
    Lane_departure_warning=0;
    during:
    Driver_control=0;
    exit:
    Lane_departure_warning=1;
  state Lane_Departure_warning
    entry:
    Driver_Control_Lamp=1;
    LKA_Enable_Lamp=1;
    LKA_Active_Lamp=0;
    Partial_Braking=0;
    Lane_departure_warning=1;
    during:
    Driver_control=1;
  (default) -> Driver_control
  LKA_Initating -> (junction 11) [order 1] : [Lane_Strength==0]
  (junction 11) -> Driver_control : {No_Detection=1;}
  Driver_control -> LKA_Initating : [LKA_Enable==1&&Lane_Strength==1]{No_Detection=0;}
  LKA_active -> Driver_control [order 2] : [Lane_Strength==0]{No_Detection=1;}
  LKA_Initating -> Driver_control [order 2] : [LKA_Enable==0]
  LKA_Initating -> (junction 15) [order 3]
  Lane_Departure_warning -> LKA_Initating : after(1.2,sec)
  LKA_active -> Driver_control [order 1] : [LKA_Enable==0]
  (junction 15) -> LKA_active [order 1] : [L1*sin(headingangle)+Lateral_offset<(.5*lane_width)]
  (junction 15) -> (junction 20) [order 2] : [L1*sin(headingangle)+Lateral_offset>(.5*lane_width)]
  LKA_active -> (junction 20) [order 3] : [abs(lateral_acc)>threshold_L_acc]
  (junction 20) -> (junction 24) [order 1] : [Lateral_offset<0]
  (junction 20) -> (junction 25) [order 2]
  (junction 24) -> (junction 27) : {Left_lane_change_lamp=1;}
  (junction 25) -> (junction 29) [order 1] : [Lateral_offset>0]
  (junction 25) -> (junction 26) [order 2] : [Lateral_offset==0]
      | {Right_lane_change_lamp=0,
      | Left_lane_change_lamp=0;}
  (junction 29) -> (junction 28) : {Right_lane_change_lamp=1;}
  (junction 28) -> (junction 26)
  (junction 27) -> (junction 28)
  (junction 26) -> Lane_Departure_warning
  data: LKA_Active_Lamp output; Lane_departure_warning output; Partial_Braking output; Left_lane_change_lamp output; Right_lane_change_lamp output; LKA_Enable input; Lane_Strength input; Lateral_offset input; headingangle input; lane_width input; lateral_acc input; threshold_L_acc input; Driver_Control_Lamp output; Driver_control output; LKA_Enable_Lamp output; No_Detection output; L1 input
